simulink model "power_svpwm"  (Simulink 6.0)
settings: Solver=FixedStepDiscrete  SolverMode=SingleTasking  StartTime=0.0  StopTime=1.5  FixedStep=Ts  RelTol=1e-3
PreLoadFcn:
  | Ts=2e-6;load xinit_power_svpwm;
undefined symbols (not defined in the file or in its folder): DiscIntNeverNeededParam
libraries: powerlib_extras x9, powerlib x4, powerlib_models x2
settings Model: Creator=Gilber Sybille, IREQ  LastModifiedBy=batserve  ExtModeAutoUpdateStatusClock=off
settings DataIOCC: LimitDataPoints=off  LoadInitialState=on  SaveFormat=Structure  SaveOutput=off  SaveTime=off  SignalLoggingName=sigsOut
settings OptimizationCC: BooleanDataType=off
settings DebuggingCC: CheckExecutionContextPreStartOutputMsg=on  CheckExecutionContextRuntimeOutputMsg=on  SolverPrmCheckMsg=none
settings HardwareCC: TargetUnknown=on

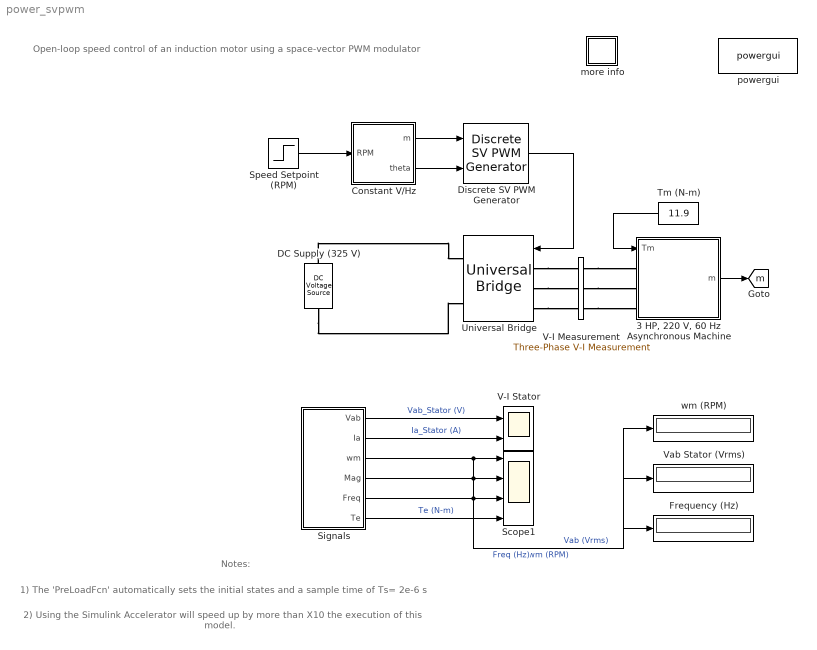
== system power_svpwm ==
  note: Open-loop speed control of an induction motor using
      | a space-vector PWM modulator
  note: 1) The 'PreLoadFcn' automatically sets
      |      the initial states and a sample time of Ts= 2e-6 s
  note: 2) Using the Simulink Accelerator will speed up by more
      |      than X10 the execution of this model.
  note: Notes:
  "3 HP, 220 V, 60 Hz Asynchronous Machine" : Subsystem  AncestorBlock=powerlib/Machines/Asynchronous Machine SI Units  mask(Asynchronous Machine){PresetModel=No, ShowDetailedParameters=on, RotorType=Squirrel-cage, ReferenceFrame=Stationary, NominalParameters=[ 3*746, 220, 60 ], Stator=[ 0.435  2*2.0e-3 ], Rotor=[ 0.816  2.0e-3 ], Lm=69.31e-3, Mechanical=[ 0.089  0  2 ], InitialConditions=[0.044533 0 11.138 11.138 11.138 -39.6 -159.6 80.4], Units=1, LoadFlowParameters=2000}
      mask prompts: PresetModel "Preset model:"; ShowDetailedParameters "-----------------  Show detailed parameters -----------------"; RotorType "Rotor type:"; ReferenceFrame "Reference frame:"; NominalParameters "Nominal power, voltage (line-line), and frequency [ Pn(VA),Vn(Vrms),fn(Hz) ]:"; Stator "Stator resistance and inductance[ Rs(ohm)  Lls(H) ]:"; Rotor "Rotor resistance and inductance [ Rr'(ohm)  Llr'(H) ]:"; Lm "Mutual inductance Lm (H):"; Mechanical "Inertia, friction factor and pairs of poles [ J(kg.m^2)  F(N.m.s)  p() ]:"; InitialConditions "Initial conditions"; Units "IOunits"; LoadFlowParameters "Load flow Parameters"
      mask help:
      | Implements a three-phase asynchronous machine (wound rotor or squirrel cage)
      | modeled in the dq rotor reference frame. Stator and rotor windings are connected
      | in wye to an internal neutral point. You can specify initial values for stator and rotor
      | currents or for  the stator current only.
      mask init:
      | block = gcb;
      | ctrl = ReferenceFrame;
      | one_third=1/3; 
      | sqrt3_3=sqrt(3)/3;
      | sqrt3=sqrt(3);
      | switch RotorType
      |     case 1, selWidth=6; elements1=3:6; elements2=1:4;
      |     case 2, selWidth=4; elements1=1:4; elements2=3:4;
      | end
      | powericon('psbloadfunction',block,'gotofrom','Initialize');
      | [NominalParameters,Stator,Rotor,Lm,Mechanical,InitialConditions] = powericon('AsynchronousMachineConvert',NominalParameters,Stator,Rotor,Lm,Mechanical,InitialConditions);	
      | Ts = powericon('AsynchronousMachineInit',block);
      | [p1,p2,p3,p4,p5,p6,p7,p8,p9,p10,p11,p12,p13,p14,p15,p16] = powericon('AsynchronousMachineIcon');
      | [Rs,Lls,Rr,Llr,H,F,p,Laq,Lad,web_psb,Vb,Vb2,ib,ib2,phib2,Nb2,Tb2,phisqo,phisdo,phirqo,phirdo,wmo,tho] = powericon('AsynchronousMachineParam',NominalParameters,Stator,Rotor,Lm,Mechanical,InitialConditions,Units);
      | powericon('AsynchronousMachineCback',block);
      settings: CopyFcn=powericon('psbloadfunction',gcbh,'gotofrom','UpdateGotoTag');
      mask Help: web(psbhelp);
      mask StyleString: popup(No|01:  5 HP   460 V 60Hz 1750 RPM           |02:  10 HP  460 V 60Hz 1760 RPM          |03:  20 HP  460 V 60Hz 1760 RPM          |04:  50 HP  460 V 60Hz 1780 RPM          |05:  100 HP 460 V 60Hz 1780 RPM         |06:  150 HP 460 V 60Hz 1785 RPM         |07:  200 HP 460 V 60Hz 1785 RPM         |08:  5 HP   575 V 60Hz 1750 RPM           |09:  10 HP  575 V 60Hz 1760 RPM          |10:  20 HP  575 V 60Hz 1765 RPM          |11:  50 HP  575 V 60Hz 1775 RPM          |12:  100 HP 575 V 60Hz 1780 RPM         |13:  150 HP 575 V 60Hz 1785 RPM         |14:  200 HP 575 V 60Hz 1785 RPM         |15:  5.4 HP (4KW)   400 V  50Hz 1430 RPM  |16:  10 HP (7.5KW)  400 V 50Hz 1440 RPM |17:  20 HP (15KW)   400 V 50Hz 1460 RPM  |18:  50 HP (37KW)   400 V 50Hz 1480 RPM  |19:  100 HP (75KW)  400 V 50Hz 1484 RPM |20:  150 HP (110KW) 400 V 50Hz 1487 RPM|21:  215 HP (160KW) 400 V 50Hz 1487 RPM),checkbox,popup(Wound|Squirrel-cage),popup(Rotor|Stationary|Synchronous),edit,edit,edit,edit,edit,edit,edit,edit
      mask CallbackString: powericon('AsynchronousMachineCback',gcb,'SI');|powericon('AsynchronousMachineCback',gcb);|powericon('AsynchronousMachineCback',gcb);|||||||||
      mask Display: plot(-55,-30,55,90,p1,p2,p3,p4,p5,p6,p7,p8,p15,p16);color('blue');plot([-30,-10,-10],[70,70,55]);
  Constant V/Hz : Subsystem
  DC Supply (325 V) : powerlib/Electrical Sources/DC Voltage Source  Orientation=up  Amplitude=325  Measurements=None
  Discrete SV PWM Generator : powerlib_extras/Discrete  Control Blocks/Discrete SV PWM Generator  InputType=Magnitude-Angle (rad)  SwitchingPattern=Pattern #1  Fc=1980  ParUref=[0.8 -30 50]  Ts=Ts
  Frequency (Hz) : Display
      settings: Format=bank  SampleTime=Ts*1000
  Scope1 : Scope  NumInputPorts=4
      settings: TimeRange=1.5  YMin=1550~219.825~59.997~-30  YMax=1585~220.05~60.0005~60  SaveName=VI_Stator1  SampleInput=on  SampleTime=Ts*100
  Signals : Subsystem
  Speed Setpoint (RPM) : Step  Time=0.1  Before=1725  After=1300  SampleTime=Ts
  Tm (N-m) : Constant  Orientation=left  Value=11.9
  Universal Bridge : powerlib/Power Electronics/Universal Bridge  Orientation=left  Arms=3  SnubberResistance=1e5  SnubberCapacitance=inf  Device=MOSFET / Diodes  Ron=0.2e-3  Lon=0  ForwardVoltages="[  0  0  ]"  ForwardVoltage=0  GTOparameters=[ 10e-6 , 20e-6 ]  IGBTparameters=[ 1e-6 , 2e-6 ]  Measurements=None
  V-I Measurement : powerlib/Measurements/Three-Phase V-I Measurement  VoltageMeasurement=phase-to-phase  SetLabelV=on  LabelV=Vabc_Stator  Vpu=off  Vbase=500e3  CurrentMeasurement=yes  SetLabelI=on  LabelI=Iabc_Stator  Ipu=off  Pbase=100e6  OutputType=Magnitude  PhasorSimulation=off  PSBequivalent=0
  V-I Stator : Scope  NumInputPorts=2
      settings: TimeRange=0.1  YMin=-400~-25  YMax=400~25  SaveName=VI_Stator  SampleInput=on  SampleTime=Ts*5
  Vab Stator (Vrms) : Display
      settings: Format=bank  SampleTime=Ts*1000
  more info : Subsystem
      mask Display: disp('?')
  powergui : powerlib/powergui  Priority=2  Frange=[0:2:500]  Ylog=off  Xlog=on  save=off  variable=ZData  structure=VI_Stator  ZoomFFT=on  StartTime=0.05  cycles=2  DisplayStyle=1  fundamental=60  FreqAxis=off  MaxFrequency=5000  frequencyindice=1  frequencyindicesteady=1  RmsSteady=1  display=off  Ts=Ts  methode=off  frequency=60  echomessages=off
  wm (RPM) : Display
      settings: SampleTime=Ts*1000
  tag scope: m=global
  wires:
  "3 HP, 220 V, 60 Hz Asynchronous Machine"/1(m) -> [m]
  Constant V/Hz/2(theta) -> Discrete SV PWM Generator/2
  Signals/1(Vab) -> V-I Stator/1  "Vab_Stator (V)"
  Signals/2(Ia) -> V-I Stator/2  "Ia_Stator (A)"
  Signals/6(Te) -> Scope1/4  "Te (N-m)"
  Constant V/Hz/1(m) -> Discrete SV PWM Generator/1
  Discrete SV PWM Generator/1 -> Universal Bridge/1
  Tm (N-m)/1 -> "3 HP, 220 V, 60 Hz Asynchronous Machine"/1(Tm)
  Signals/3(wm) -> Scope1/1, wm (RPM)/1  "wm (RPM)"
  Signals/4(Mag) -> Scope1/2, Vab Stator (Vrms)/1  "Vab (Vrms)"
  Signals/5(Freq) -> Scope1/3, Frequency (Hz)/1  "Freq (Hz)"
  Speed Setpoint (RPM)/1 -> Constant V/Hz/1(RPM)
  connections:
  DC Supply (325 V)/RConn1 -- Universal Bridge/RConn1
  DC Supply (325 V)/LConn1 -- Universal Bridge/RConn2
  Universal Bridge/LConn1 -- V-I Measurement/LConn1
  Universal Bridge/LConn2 -- V-I Measurement/LConn2
  Universal Bridge/LConn3 -- V-I Measurement/LConn3
  V-I Measurement/RConn1 -- "3 HP, 220 V, 60 Hz Asynchronous Machine"/LConn1
  V-I Measurement/RConn2 -- "3 HP, 220 V, 60 Hz Asynchronous Machine"/LConn2
  V-I Measurement/RConn3 -- "3 HP, 220 V, 60 Hz Asynchronous Machine"/LConn3

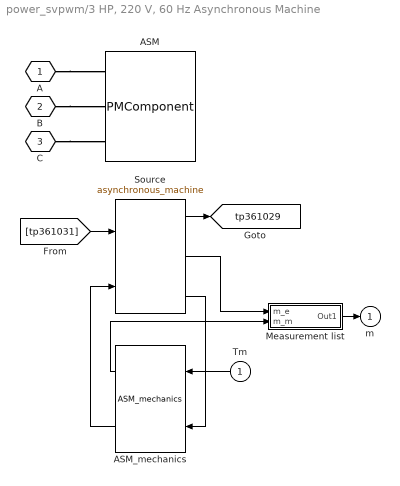
== system power_svpwm/3 HP, 220 V, 60 Hz Asynchronous Machine ==
  Tm : Inport  Orientation=left  Port=1  LatchInput=off
  ASM : PMComponent  PhysicalDomain=powersysdomain  LeftPortType=p1  RightPortType=p1  LConnTagsString=A|B|C  RConnTagsString=a|b|c
      mask Type: InnerPowersysBlock
  ASM_mechanics : powerlib_models/Discrete/ASM_mechanics  Orientation=left
  Measurement list : Subsystem
  Source : powerlib_models/Discrete/asynchronous_machine
  A : PMIOPort  Port=1  Side=Left
  B : PMIOPort  Port=2  Side=Left
  C : PMIOPort  Port=3  Side=Left
  m : Outport  InitialOutput=0
  tag scope: tp361029=global
  wires:
  ASM_mechanics/1 -> Measurement list/2(m_m)
  Source/2 -> Measurement list/1(m_e)
  ASM_mechanics/2 -> Source/2
  [tp361031] -> Source/1
  Source/1 -> [tp361029]
  Source/3 -> ASM_mechanics/2
  Tm/1 -> ASM_mechanics/1
  Measurement list/1(Out1) -> m/1
  connections:
  A/RConn1 -- ASM/LConn1
  B/RConn1 -- ASM/LConn2
  C/RConn1 -- ASM/LConn3

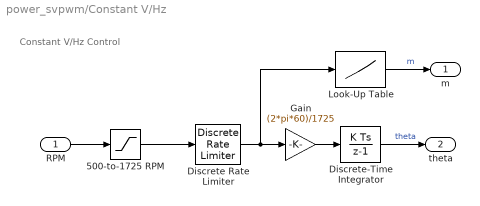
== system power_svpwm/Constant V/Hz ==
  note: Constant V/Hz
      | Control
  RPM : Inport  Port=1  LatchInput=off
  500-to-1725 RPM : Saturate  UpperLimit=1725  LowerLimit=500
  Discrete Rate Limiter : powerlib_extras/Discrete  Control Blocks/Discrete Rate Limiter  R=500  F=-500  Vinit=1725  Ts=Ts
  Discrete-Time Integrator : DiscreteIntegrator  SampleTime=Ts  ICPrevOutput=DiscIntNeverNeededParam  ICPrevScaledInput=DiscIntNeverNeededParam
  Gain : Gain  Gain=(2*pi*60)/1725  SaturateOnIntegerOverflow=on
  Look-Up Table : Lookup  DialogController=Simulink.DDGSource  InputValues=[500 1725 2500]  OutputValues=[0.29 1 1]*0.957  SaturateOnIntegerOverflow=on
  m : Outport
  theta : Outport  Port=2
  wires:
  Gain/1 -> Discrete-Time Integrator/1
  Discrete Rate Limiter/1 -> Gain/1, Look-Up Table/1
  Look-Up Table/1 -> m/1  "m"
  RPM/1 -> 500-to-1725 RPM/1
  Discrete-Time Integrator/1 -> theta/1  "theta"
  500-to-1725 RPM/1 -> Discrete Rate Limiter/1

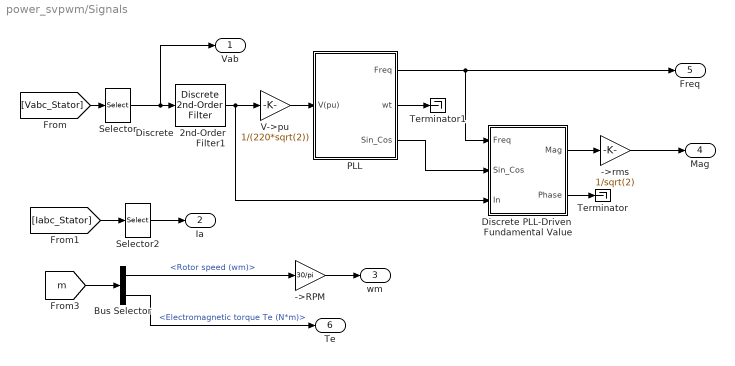
== system power_svpwm/Signals ==
  ->RPM : Gain  Gain=30/pi  SaturateOnIntegerOverflow=on
  ->rms : Gain  Gain=1/sqrt(2)  SaturateOnIntegerOverflow=on
  Bus Selector : BusSelector  DialogController=Simulink.DDGSource_Bus  OutputSignals=Mechanical.Rotor speed (wm),Mechanical.Electromagnetic torque Te (N*m)
  Discrete PLL-Driven  Fundamental Value : Subsystem  mask(Discrete PLL-Driven Fundamental Value){Finit=60, Par_Init=[220*sqrt(2) 0], Ts=Ts*20}
      mask prompts: Finit "Initial fundamental frequency (Hz):"; Par_Init "Initial input: [ Mag  Phase-relative-to-PLL(degrees) ]"; Ts "Sample time:"
      mask help:
      | This discrete block computes the fundamental value of the input signal (port In) over a running window of one cycle of a specified fundamental frequency (port Freq). Input port "Sin_Cos" (a two-dimension signal) provides the reference frame required for the computation..
      |  First and second outputs return respectively the magnitude and phase (in degrees relative to the PLL phase) of the fundamental.
      | For the first cycle of simulation, the ouputs are held constant to the values specified by the parameter "Initial input".
      mask init:
      | Real_Init=Par_Init(1)*cos(pi/180*Par_Init(2));
      | Imag_Init=Par_Init(1)*sin(pi/180*Par_Init(2));
  Discrete  2nd-Order Filter1 : powerlib_extras/Discrete  Control Blocks/Discrete  2nd-Order Filter  FilterType=Lowpass  Fo=2000  Zeta=0.707  Ts=Ts  Initialize=on  Vac_Init=[1 30 60]  Vdc_Init=0  PlotResponse=off  param1=[1 500 1]
  PLL : Subsystem  mask(Discrete 1-phase PLL){Par_Init=[27.52 60], ParK=[120 2800], Ts=Ts*20}
      mask prompts: Par_Init "Initial input:[ Phase(degrees)   Frequency(Hz) ]"; ParK "Regulator gains [ Kp  Ki ]"; Ts "Sample time:"
      mask help:
      | This Phase Locked Loop (PLL) system can be used  to synchronize on a variable frequency sinusoidal signal.
      |
      | Input 1: Normalized input signal V(pu)
      |
      | Output 1:  Measured frequency (Hz) = w/(2pi)
      | Output 2:  Ramp w.t  varying between  0 and 2*pi, synchronized on the zero-crossing (rising) of  the input signal
      | Output 3: Vector [sin(wt) cos(wt)]
      mask init:
      | Kp=ParK(1);
      | Ki=ParK(2);
      | Phase_Init=Par_Init(1);
      | Finit=Par_Init(2);
  Selector : Selector  Elements=[1]  InputPortWidth=3
  Selector2 : Selector  Elements=[1]  InputPortWidth=3
  Terminator : Terminator
  Terminator1 : Terminator
  V->pu : Gain  Gain=1/(220*sqrt(2))  SaturateOnIntegerOverflow=on
  Vab : Outport
  Ia : Outport  Port=2
  wm : Outport  Port=3
  Mag : Outport  Port=4
  Freq : Outport  Port=5
  Te : Outport  Port=6
  wires:
  PLL/2(wt) -> Terminator1/1
  PLL/3(Sin_Cos) -> Discrete PLL-Driven  Fundamental Value/2(Sin_Cos)
  V->pu/1 -> PLL/1(V(pu))
  Selector/1 -> Vab/1, Discrete  2nd-Order Filter1/1
  Discrete PLL-Driven  Fundamental Value/1(Mag) -> ->rms/1
  [Vabc_Stator] -> Selector/1
  [Iabc_Stator] -> Selector2/1
  ->RPM/1 -> wm/1
  ->rms/1 -> Mag/1
  Selector2/1 -> Ia/1
  Discrete  2nd-Order Filter1/1 -> V->pu/1, Discrete PLL-Driven  Fundamental Value/3(In)
  [m] -> Bus Selector/1
  Bus Selector/1 -> ->RPM/1  "<Rotor speed (wm)>"
  Bus Selector/2 -> Te/1  "<Electromagnetic torque Te (N*m)>"
  PLL/1(Freq) -> Discrete PLL-Driven  Fundamental Value/1(Freq), Freq/1
  Discrete PLL-Driven  Fundamental Value/2(Phase) -> Terminator/1

== system power_svpwm/more info ==
  note: Louis-A. Dessaint and R. Champagne (Ecole de Technologie Superieure, Montreal)
  note: Start the simulation. Since the initial states values have been automatically loaded, the simulation should start in steady-state.
      | The initial motor speed should be 1720 RPM and the rms value of the stator voltages should be 220V@60Hz.
      |
      | At 0.1s, the speed setpoint is changed from 1725 to 1300 RPM.  You can observe the system dynamic looking inside
      | Scope 1. When the motor reaches a constant speed of 1275 RPM, the stator voltage rms value is down to 165.8V and
      | the frequency to 45.2 Hz.
      |
      | Stator voltage (phase AB) and phase A current waveforms can be observed in the "V-I Stator" Scope. You can do a FFT
      | of theses two quantities using the powergui FFT Analysis.
  note: Open-loop speed control of an induction motor using constant V/Hz principle and SV PWM technique
  note: Circuit Description
  note: Demonstration
  note: A 3-phase squirrel-cage motor rated 3 HP, 220 V, 60 Hz, 1725 rpm is fed by a 3-phase MOSFET inverter connected
      | to a DC voltage source of 325 V. The inverter is modeled using the "Universal Bridge" block and the motor by the
      | "Asynchronous Machine" block. Its stator leakage inductance Lls is set to twice its actual value to simulate the effect of a
      | smoothing reactor placed between the inverter  and the machine. The load torque applied to the  machine's shaft is
      | constant and set to its nominal value of 11.9 N.m.
      |
      | The firing pulses to the inverter are generated  by the "Space-Vector PWM modulator" block of the SPS library.
      | The chopping frequency is set to 1980 Hz and the input reference vector to "Magnitude-Angle".
      |
      | Speed control of the motor is performed by the "Constant V/Hz" block.  The magnitude and frequency of the stator voltages
      | are set based on the speed setpoint. By varying the stator voltages magnitude in proportion with frequency, the stator flux is
      | kept constant.

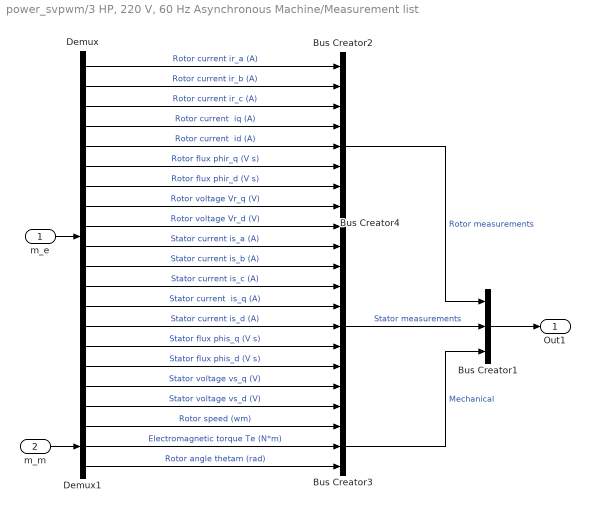
== system power_svpwm/3 HP, 220 V, 60 Hz Asynchronous Machine/Measurement list ==
  m_e : Inport  Port=1  LatchInput=off
  m_m : Inport  Port=2  LatchInput=off
  Bus Creator1 : BusCreator  DialogController=Simulink.DDGSource_Bus  Inputs=3
  Bus Creator2 : BusCreator  DialogController=Simulink.DDGSource_Bus  Inputs=9
  Bus Creator3 : BusCreator  DialogController=Simulink.DDGSource_Bus  Inputs=3
  Bus Creator4 : BusCreator  DialogController=Simulink.DDGSource_Bus  Inputs=9
  Demux : Demux  Outputs=[1,1,1,1,1,1,1,1,1,1,1,1,1,1,1,1,1,1]
  Demux1 : Demux  Outputs=[1,1,1]
  Out1 : Outport
  wires:
  m_m/1 -> Demux1/1
  m_e/1 -> Demux/1
  Bus Creator1/1 -> Out1/1
  Demux/1 -> Bus Creator2/1  "Rotor current ir_a (A)"
  Demux/2 -> Bus Creator2/2  "Rotor current ir_b (A)"
  Demux/3 -> Bus Creator2/3  "Rotor current ir_c (A)"
  Bus Creator2/1 -> Bus Creator1/1  "Rotor measurements"
  Demux/4 -> Bus Creator2/4  "Rotor current  iq (A)"
  Demux/5 -> Bus Creator2/5  "Rotor current  id (A)"
  Demux/6 -> Bus Creator2/6  "Rotor flux phir_q (V s)"
  Demux/7 -> Bus Creator2/7  "Rotor flux phir_d (V s)"
  Demux/8 -> Bus Creator2/8  "Rotor voltage Vr_q (V)"
  Demux/9 -> Bus Creator2/9  "Rotor voltage Vr_d (V)"
  Demux/10 -> Bus Creator4/1  "Stator current is_a (A)"
  Demux/11 -> Bus Creator4/2  "Stator current is_b (A)"
  Demux/12 -> Bus Creator4/3  "Stator current is_c (A)"
  Demux/13 -> Bus Creator4/4  "Stator current  is_q (A)"
  Demux/14 -> Bus Creator4/5  "Stator current is_d (A)"
  Bus Creator4/1 -> Bus Creator1/2  "Stator measurements"
  Demux1/3 -> Bus Creator3/3  "Rotor angle thetam (rad)"
  Demux1/2 -> Bus Creator3/2  "Electromagnetic torque Te (N*m)"
  Demux1/1 -> Bus Creator3/1  "Rotor speed (wm)"
  Demux/15 -> Bus Creator4/6  "Stator flux phis_q (V s)"
  Demux/16 -> Bus Creator4/7  "Stator flux phis_d (V s)"
  Demux/17 -> Bus Creator4/8  "Stator voltage vs_q (V)"
  Demux/18 -> Bus Creator4/9  "Stator voltage vs_d (V)"
  Bus Creator3/1 -> Bus Creator1/3  "Mechanical"

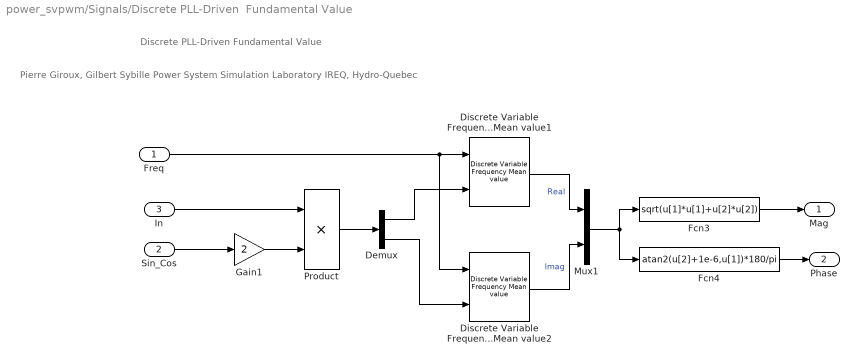
== system power_svpwm/Signals/Discrete PLL-Driven  Fundamental Value ==
  note: Discrete PLL-Driven Fundamental Value
  note: Pierre Giroux, Gilbert Sybille
      | Power System Simulation Laboratory
      | IREQ, Hydro-Quebec
  Freq : Inport  Port=1  LatchInput=off
  Sin_Cos : Inport  Port=2  LatchInput=off
  In : Inport  Port=3  LatchInput=off
  Demux : Demux  Outputs=2
  Discrete Variable Frequency Mean value1 : powerlib_extras/Discrete Measurements/Discrete Variable Frequency Mean value  Finit=Finit  Fmin=20  Vinit=Real_Init  Ts=Ts
  Discrete Variable Frequency Mean value2 : powerlib_extras/Discrete Measurements/Discrete Variable Frequency Mean value  Finit=Finit  Fmin=20  Vinit=Imag_Init  Ts=Ts
  Fcn3 : Fcn  Expr=sqrt(u[1]*u[1]+u[2]*u[2])
  Fcn4 : Fcn  Expr=atan2(u[2]+1e-6,u[1])*180/pi
  Gain1 : Gain  Gain=2  SaturateOnIntegerOverflow=on
  Mux1 : Mux  Inputs=2
  Product : Product  SaturateOnIntegerOverflow=on  InputSameDT=on
  Mag : Outport
  Phase : Outport  Port=2
  wires:
  Mux1/1 -> Fcn3/1, Fcn4/1
  Fcn3/1 -> Mag/1
  Fcn4/1 -> Phase/1
  Discrete Variable Frequency Mean value2/1 -> Mux1/2  "Imag"
  Discrete Variable Frequency Mean value1/1 -> Mux1/1  "Real"
  Demux/1 -> Discrete Variable Frequency Mean value1/2
  Gain1/1 -> Product/2
  Product/1 -> Demux/1
  Demux/2 -> Discrete Variable Frequency Mean value2/2
  Freq/1 -> Discrete Variable Frequency Mean value2/1, Discrete Variable Frequency Mean value1/1
  Sin_Cos/1 -> Gain1/1
  In/1 -> Product/1

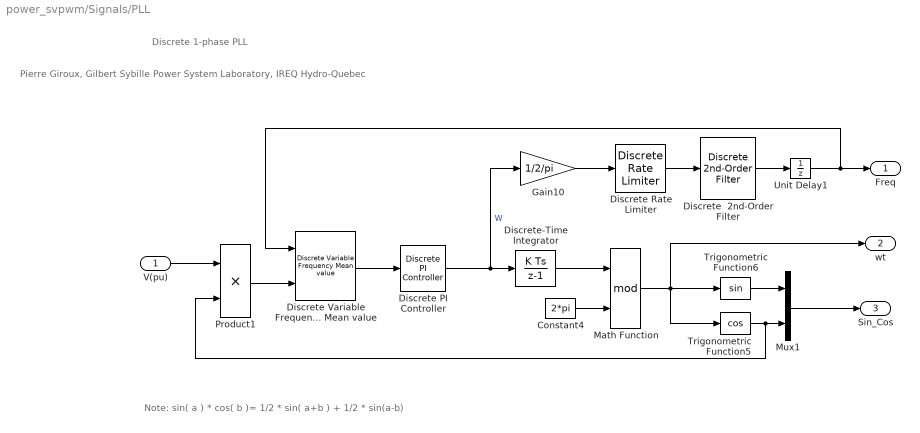
== system power_svpwm/Signals/PLL ==
  note: Pierre Giroux, Gilbert Sybille
      | Power System Laboratory, IREQ
      | Hydro-Quebec
  note: Note: sin( a ) * cos( b )= 1/2 * sin( a+b ) + 1/2 * sin(a-b)
  note: Discrete 1-phase PLL
  V(pu) : Inport  Port=1  LatchInput=off
  Constant4 : Constant  Value=2*pi
  Discrete PI Controller : powerlib_extras/Discrete  Control Blocks/Discrete PI Controller  Kp=Kp  Ki=Ki  Par_Limits="[4  0.25]*2*pi*Finit"  Init=2*pi*Finit  Ts=Ts
  Discrete Rate Limiter : powerlib_extras/Discrete  Control Blocks/Discrete Rate Limiter  R=30  F=-30  Vinit=Finit  Ts=Ts
  Discrete Variable Frequency Mean value : powerlib_extras/Discrete Measurements/Discrete Variable Frequency Mean value  Finit=Finit  Fmin=10  Vinit=0  Ts=Ts
  Discrete  2nd-Order Filter : powerlib_extras/Discrete  Control Blocks/Discrete  2nd-Order Filter  FilterType=Lowpass  Fo=25  Zeta=0.707  Ts=Ts  Initialize=on  Vac_Init="[0 0  Finit]"  Vdc_Init=Finit  PlotResponse=off  param1=[1 500 0.1]
  Discrete-Time Integrator : DiscreteIntegrator  InitialCondition=Phase_Init*pi/180  SampleTime=Ts  UpperSaturationLimit=0  LowerSaturationLimit=0  ICPrevOutput=DiscIntNeverNeededParam  ICPrevScaledInput=DiscIntNeverNeededParam
  Gain10 : Gain  Gain=1/2/pi  SaturateOnIntegerOverflow=on
  Math Function : Math  Operator=mod  SaturateOnIntegerOverflow=on
  Mux1 : Mux  Inputs=2
  Product1 : Product  SaturateOnIntegerOverflow=on  InputSameDT=on
  Trigonometric Function5 : Trigonometry  Operator=cos
  Trigonometric Function6 : Trigonometry
  Unit Delay1 : UnitDelay  X0=Finit  SampleTime=Ts
  Freq : Outport
  wt : Outport  Port=2
  Sin_Cos : Outport  Port=3
  wires:
  Unit Delay1/1 -> Discrete Variable Frequency Mean value/1, Freq/1
  Discrete PI Controller/1 -> Gain10/1, Discrete-Time Integrator/1  "W"
  V(pu)/1 -> Product1/1
  Constant4/1 -> Math Function/2
  Discrete-Time Integrator/1 -> Math Function/1
  Product1/1 -> Discrete Variable Frequency Mean value/2
  Discrete Variable Frequency Mean value/1 -> Discrete PI Controller/1
  Mux1/1 -> Sin_Cos/1
  Math Function/1 -> Trigonometric Function6/1, Trigonometric Function5/1, wt/1
  Trigonometric Function6/1 -> Mux1/1
  Trigonometric Function5/1 -> Mux1/2, Product1/2
  Discrete  2nd-Order Filter/1 -> Unit Delay1/1
  Gain10/1 -> Discrete Rate Limiter/1
  Discrete Rate Limiter/1 -> Discrete  2nd-Order Filter/1
